simulink model "sim12b"  (R2015a)
settings: Solver=ode45  StartTime=0.0  StopTime=10.0  RelTol=1e-3
values from neighbouring files (symbols this model uses):
  b = 0    [lab2.m]
  k1 = 1/yl    (= 20)    [lab2.m]
  k2 = sqrt(2*k1)    [lab2.m]
  yl = 0.05    [lab2.m]
undefined symbols (not defined in the file or in its folder): sgn
libraries: simulink x2
settings Model: Creator=Pedro  LastModifiedBy=Pedro

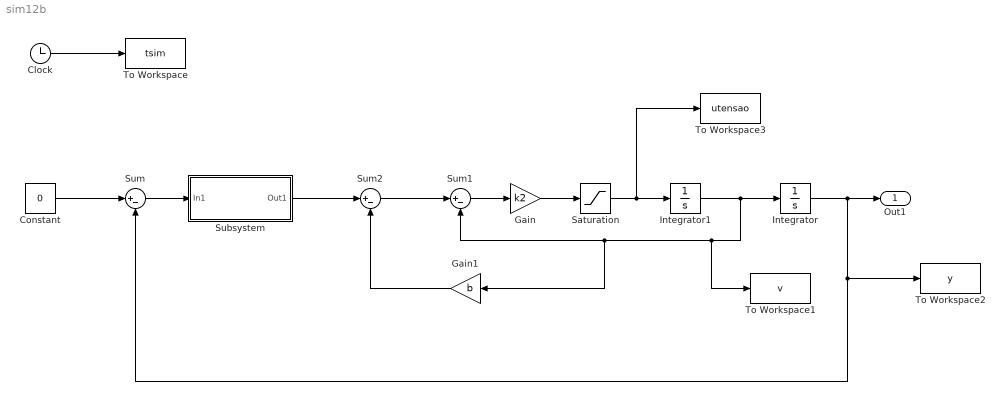
== system sim12b ==
  Clock : Clock
  Constant : Constant  Value=0
  Gain : Gain  Gain=k2
  Gain1 : Gain  Gain=b
  Integrator : Integrator  InitialCondition=1
  Integrator1 : Integrator
  Saturation : Saturate  UpperLimit=1  LowerLimit=-1
  Subsystem : Subsystem
  Sum : Sum  Inputs=|+-
  Sum1 : Sum  Inputs=|+-
  Sum2 : Sum  Inputs=|+-
  To Workspace : ToWorkspace  VariableName=tsim  SampleTime=-1
  To Workspace1 : ToWorkspace  VariableName=v  SampleTime=-1
  To Workspace2 : ToWorkspace  VariableName=y  SampleTime=-1
  To Workspace3 : ToWorkspace  VariableName=utensao  SampleTime=-1
  Out1 : Outport
  wires:
  Sum1/1 -> Gain/1
  Gain/1 -> Saturation/1
  Saturation/1 -> To Workspace3/1, Integrator1/1
  Integrator1/1 -> To Workspace1/1, Gain1/1, Sum1/2, Integrator/1
  Constant/1 -> Sum/1
  Integrator/1 -> To Workspace2/1, Sum/2, Out1/1
  Clock/1 -> To Workspace/1
  Sum/1 -> Subsystem/1(In1)
  Sum2/1 -> Sum1/1
  Subsystem/1(Out1) -> Sum2/1
  Gain1/1 -> Sum2/2

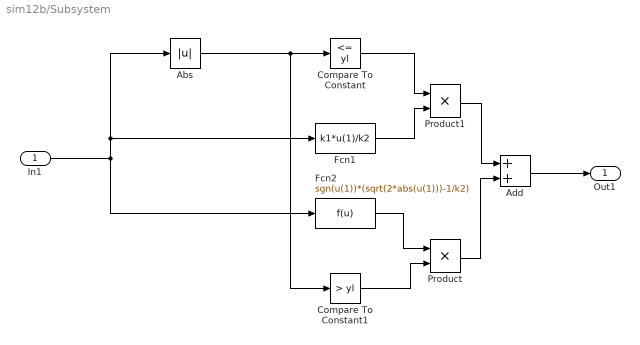
== system sim12b/Subsystem ==
  In1 : Inport
  Abs : Abs
  Add : Sum
  Compare To Constant : simulink/Logic and Bit Operations/Compare To Constant  relop=<=  const=yl  OutDataTypeStr=boolean
  Compare To Constant1 : simulink/Logic and Bit Operations/Compare To Constant  relop=>  const=yl  OutDataTypeStr=boolean
  Fcn1 : Fcn  Expr=k1*u(1)/k2
  Fcn2 : Fcn  Expr=sgn(u(1))*(sqrt(2*abs(u(1)))-1/k2)
  Product : Product
  Product1 : Product
  Out1 : Outport
  wires:
  Product/1 -> Add/2
  Product1/1 -> Add/1
  Compare To Constant/1 -> Product1/1
  Abs/1 -> Compare To Constant1/1, Compare To Constant/1
  Fcn1/1 -> Product1/2
  Fcn2/1 -> Product/1
  Compare To Constant1/1 -> Product/2
  Add/1 -> Out1/1
  In1/1 -> Fcn2/1, Fcn1/1, Abs/1
